simulink model "SlotineAdaptableMotor"  (Simulink 6.6)
settings: Solver=ode1  SolverMode=SingleTasking  StartTime=0.0  StopTime=10  FixedStep=0.001  RelTol=1e-3
values from neighbouring files (symbols this model uses):
  alpha = 100    [datos.mat]
  Gamma = [0.5 0.5]    [datos.mat]
  kd = 0.5    [datos.mat]
  lambda = 1    [datos.mat]
libraries: Plantilla_Servo_2014 x1
settings Model: Creator=usuario  LastModifiedBy=usuario  SimulationMode=external  ExtModeArmWhenConnect=off  BufferReuse=off
settings OptimizationCC: BooleanDataType=off  InlineInvariantSignals=on  OptimizeBlockIOStorage=off  BufferReuse=off  ExpressionFolding=off  LocalBlockOutputs=off
settings RTWCC: SystemTargetFile=wincon.tlc  MakeCommand=make_wc  TemplateMakefile=wc_default_tmf  Description=WinCon Target  ProcessScript=wincon_make_rtw_hook
settings STFCustomTargetCC: TargetFcnLib=ansi_tfl_tmw.mat  GenFloatMathFcnCalls=ANSI_C  ModelReferenceCompliant=off  SystemTargetFile=wincon.tlc
settings GRTTargetCC: ModelReferenceCompliant=off  MatFileLogging=off  ExtMode=on  ExtModeMexFile=wc_comm
settings CustomProperty: Value=on

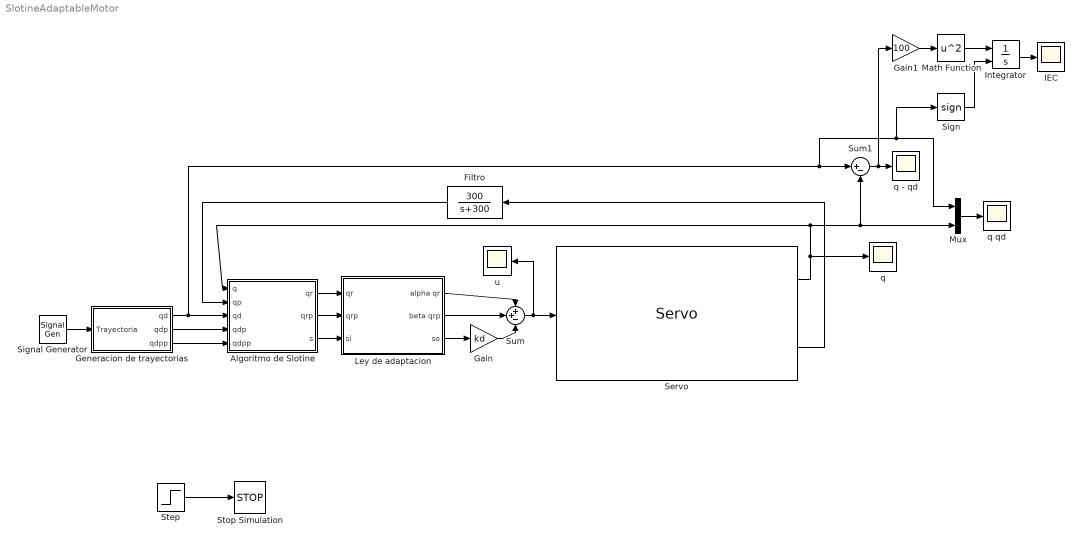
== system SlotineAdaptableMotor ==
  Algoritmo de Slotine : Subsystem
  Filtro : TransferFcn  Orientation=left  Numerator=[300]  Denominator=[1 300]
  Gain : Gain  Gain=kd
  Gain1 : Gain  Gain=100
  Generacion de trayectorias : Subsystem
  IEC : Scope
      settings: SaveName=ScopeData9
  Integrator : Integrator  ExternalReset=rising
  Ley de adaptacion : Subsystem
  Math Function : Math  Operator=square  SaturateOnIntegerOverflow=on
  Mux : Mux  Inputs=2
  Servo : Plantilla_Servo_2014/Servo  SystemSampleTime=-1
  Sign : Signum
  Signal Generator : SignalGenerator  Amplitude=0.5  Frequency=0.5
  Step : Step  Time=10  SampleTime=0
  Stop Simulation : Stop
  Sum : Sum  Inputs=++-
  Sum1 : Sum  Inputs=|+-
  q : Scope
      settings: SaveName=ScopeData8
  q - qd : Scope
      settings: SaveName=ScopeData2
  q qd : Scope
      settings: SaveName=ScopeData4
  u : Scope
      settings: SaveName=ScopeData3
  wires:
  Signal Generator/1 -> Generacion de trayectorias/1(Trayectoria)
  Generacion de trayectorias/1(qd) -> Algoritmo de Slotine/3(qd), Sum1/1, Mux/1, Sign/1
  Generacion de trayectorias/2(qdp) -> Algoritmo de Slotine/4(qdp)
  Generacion de trayectorias/3(qdpp) -> Algoritmo de Slotine/5(qdpp)
  Algoritmo de Slotine/3(s) -> Ley de adaptacion/3(si)
  Algoritmo de Slotine/2(qrp) -> Ley de adaptacion/2(qrp)
  Algoritmo de Slotine/1(qr) -> Ley de adaptacion/1(qr)
  Ley de adaptacion/3(so) -> Gain/1
  Ley de adaptacion/2(beta qrp) -> Sum/2
  Gain/1 -> Sum/3
  Ley de adaptacion/1(alpha qr) -> Sum/1
  Sum/1 -> u/1, Servo/1
  Sum1/1 -> q - qd/1, Gain1/1
  Servo/1 -> Algoritmo de Slotine/1(q), Sum1/2, Mux/2, q/1
  Servo/2 -> Filtro/1
  Filtro/1 -> Algoritmo de Slotine/2(qp)
  Mux/1 -> q qd/1
  Step/1 -> Stop Simulation/1
  Gain1/1 -> Math Function/1
  Math Function/1 -> Integrator/1
  Sign/1 -> Integrator/2
  Integrator/1 -> IEC/1

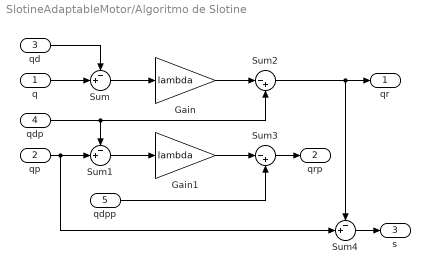
== system SlotineAdaptableMotor/Algoritmo de Slotine ==
  q : Inport
  qp : Inport  Port=2
  qd : Inport  Port=3
  qdp : Inport  Port=4
  qdpp : Inport  Port=5
  Gain : Gain  Gain=lambda
  Gain1 : Gain  Gain=lambda
  Sum : Sum  Inputs=-+|
  Sum1 : Sum  Inputs=-+|
  Sum2 : Sum  Inputs=|-+
  Sum3 : Sum  Inputs=|-+
  Sum4 : Sum  Inputs=-+|
  qr : Outport
  qrp : Outport  Port=2
  s : Outport  Port=3
  wires:
  Sum/1 -> Gain/1
  Sum1/1 -> Gain1/1
  Gain1/1 -> Sum3/1
  Gain/1 -> Sum2/1
  qd/1 -> Sum/1
  q/1 -> Sum/2
  Sum2/1 -> qr/1, Sum4/1
  qp/1 -> Sum1/2, Sum4/2
  Sum3/1 -> qrp/1
  Sum4/1 -> s/1
  qdp/1 -> Sum2/2, Sum1/1
  qdpp/1 -> Sum3/2

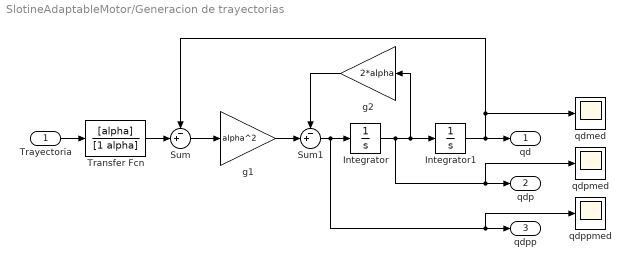
== system SlotineAdaptableMotor/Generacion de trayectorias ==
  Trayectoria : Inport
  Integrator : Integrator
  Integrator1 : Integrator
  Sum : Sum  Inputs=-+|
  Sum1 : Sum  Inputs=-+|
  Transfer Fcn : TransferFcn  Numerator=[alpha]  Denominator=[1 alpha]
  g1 : Gain  Gain=alpha^2
  g2 : Gain  Orientation=left  Gain=2*alpha
  qdmed : Scope
      settings: SaveName=ScopeData5
  qdpmed : Scope
      settings: SaveName=ScopeData6
  qdppmed : Scope
      settings: SaveName=ScopeData7
  qd : Outport
  qdp : Outport  Port=2
  qdpp : Outport  Port=3
  wires:
  Transfer Fcn/1 -> Sum/2
  Sum/1 -> g1/1
  g1/1 -> Sum1/2
  Sum1/1 -> Integrator/1, qdpp/1, qdppmed/1
  Integrator/1 -> Integrator1/1, g2/1, qdp/1, qdpmed/1
  g2/1 -> Sum1/1
  Integrator1/1 -> qd/1, Sum/1, qdmed/1
  Trayectoria/1 -> Transfer Fcn/1

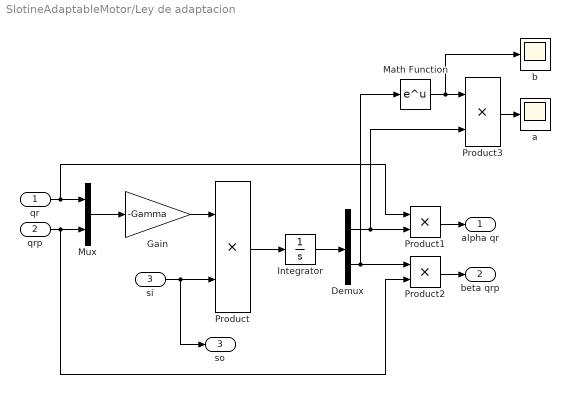
== system SlotineAdaptableMotor/Ley de adaptacion ==
  qr : Inport
  qrp : Inport  Port=2
  si : Inport  Port=3
  Demux : Demux  Outputs=2
  Gain : Gain  Gain=-Gamma
  Integrator : Integrator
  Math Function : Math  SaturateOnIntegerOverflow=on
  Mux : Mux  Inputs=2
  Product{,1..3} (4 alike) : Product  RndMeth=Zero
  a : Scope
  b : Scope
  alpha qr : Outport
  beta qrp : Outport  Port=2
  so : Outport  Port=3
  wires:
  Gain/1 -> Product/1
  Mux/1 -> Gain/1
  Product/1 -> Integrator/1
  Integrator/1 -> Demux/1
  Demux/1 -> Product1/2, Product3/2
  Demux/2 -> Product2/1, Math Function/1
  Math Function/1 -> Product3/1, b/1
  Product3/1 -> a/1
  qr/1 -> Mux/1, Product1/1
  qrp/1 -> Mux/2, Product2/2
  Product1/1 -> alpha qr/1
  Product2/1 -> beta qrp/1
  si/1 -> Product/2, so/1
